simulink model "ramp06"  (Simulink 10.0)
settings: Solver=VariableStepAuto  StartTime=0.0  StopTime=50  FixedStep=1/1000  RelTol=1e-3
model workspace (MAT data in the model file):
  A = [1  -0.0098; 0  1]
  B = [0.001; 0]
  P0 = [1000000  0; 0  1000000]
  P1 = [1000000  0  0  0  0  0  0  0  0  0  0  0  0  0  0  0  0  0  0  0; 0  1000000  0  0  0  0  0  0  0  0  0  0  0  0  0  0  0  0  0  0; 0  0  1000000  0  0  0  0  0  0  0  0  0  0  0  0  0  0  0  0  0; 0  0  0  1000000  0  0  0  0  0  0  0  0  0  0  0  0  0  0  0  0; 0  0  0  0  1000000  0  0  0  0  0  0  0  0  0  0  0  0  0  0  0; 0  0  0  0  0  1000000  0  0  0  0  0  0  0  0  0  0  0  0  0  0; 0  0  0  0  0  0  1000000  0  0  0  0  0  0  0  0  0  0  0  0  0; 0  0  0  0  0  0  0  1000000  0  0  0  0  0  0  0  0  0  0  0  0; 0  0  0  0  0  0  0  0  1000000  0  0  0  0  0  0  0  0  0  0  0; 0  0  0  0  0  0  0  0  0  1000000  0  0  0  0  0  0  0  0  0  0; 0  0  0  0  0  0  0  0  0  0  1000000  0  0  0  0  0  0  0  0  0; 0  0  0  0  0  0  0  0  0  0  0  1000000  0  0  0  0  0  0  0  0; 0  0  0  0  0  0  0  0  0  0  0  0  1000000  0  0  0  0  0  0  0; 0  0  0  0  0  0  0  0  0  0  0  0  0  1000000  0  0  0  0  0  0; 0  0  0  0  0  0  0  0  0  0  0  0  0  0  1000000  0  0  0  0  0; 0  0  0  0  0  0  0  0  0  0  0  0  0  0  0  1000000  0  0  0  0; 0  0  0  0  0  0  0  0  0  0  0  0  0  0  0  0  1000000  0  0  0; 0  0  0  0  0  0  0  0  0  0  0  0  0  0  0  0  0  1000000  0  0; 0  0  0  0  0  0  0  0  0  0  0  0  0  0  0  0  0  0  1000000  0; 0  0  0  0  0  0  0  0  0  0  0  0  0  0  0  0  0  0  0  1000000]
  P2 = 1000000
  X0 = [14; 0]
  dett = 0.001
  f = 0.0038
  g : num (value not decoded)
libraries: simulink x1, Solver_SF x1
settings Model: Creator=JHD  LastModifiedBy=JHD  OrderedModelArguments=off
settings DataIOCC: SaveFormat=Dataset  ReturnWorkspaceOutputs=on
settings OptimizationCC: LifeSpan=auto
settings DebuggingCC: UnderspecifiedInitializationDetection=Simplified  MergeDetectMultiDrivingBlocksExec=error  SFUnexpectedBacktrackingDiag=error  SFNoUnconditionalDefaultTransitionDiag=error  SFExecutionAtInitializationDiag=warning  ArithmeticOperatorsInVariantConditions=error
settings HardwareCC: ProdBitPerPointer=64  ProdBitPerSizeT=64  ProdBitPerPtrDiffT=64  ProdLargestAtomicFloat=Float  ProdIntDivRoundTo=Zero  ProdEndianess=LittleEndian  ProdWordSize=64  ProdHWDeviceType=Intel->x86-64 (Windows64)
settings ModelReferenceCC: PropagateSignalLabelsOutOfModel=on
settings SFSimCC: SimUseLocalCustomCode=on  CustomCodeUndefinedFunction=FilterOut
settings RTWCC: RTWUseLocalCustomCode=on
settings CodeAppCC: StateflowObjectComments=off
settings GRTTargetCC: TargetLangStandard=C99 (ISO)  CombineOutputUpdateFcns=on  GRTInterface=off
settings ConfigComp: CovMetricSettings=dwe  CovHtmlReporting=off  CovSaveCumulativeToWorkspaceVar=off  CovSaveSingleToWorkspaceVar=off

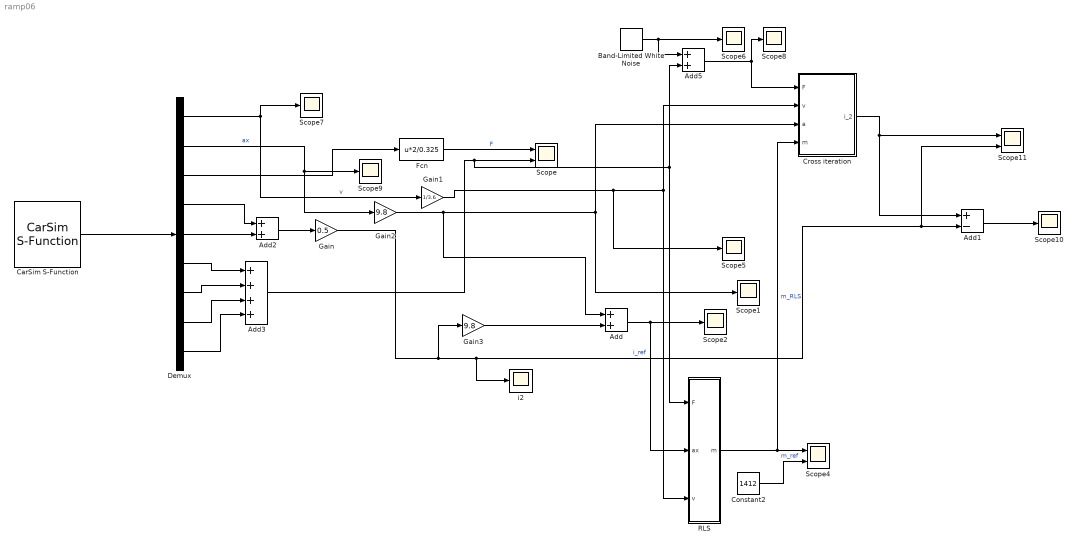
== system ramp06 ==
  Add : Sum
  Add1 : Sum  Inputs=+-
  Add2 : Sum
  Add3 : Sum  Inputs=4
  Add5 : Sum
  Band-Limited White Noise : simulink/Sources/Band-Limited White Noise  Cov=[10]  Ts=0.1  seed=[23341]
  CarSim S-Function : Solver_SF/CarSim S-Function  Priority=1  SIMFILE=simfile.sim
  Constant2 : Constant  Value=1412
  Cross iteration : Subsystem
  Demux : Demux  Outputs=9
  Fcn : Fcn  Expr=u*2/0.325
  Gain : Gain  Gain=0.5
  Gain1 : Gain  Gain=1/3.6
  Gain2 : Gain  Gain=9.8
  Gain3 : Gain  Gain=9.8
  RLS : Subsystem
  Scope : Scope  NumInputPorts=2
  Scope{1..2,5..10} (8 alike) : Scope
  Scope11 : Scope  NumInputPorts=2
  Scope4 : Scope  NumInputPorts=2
  i2 : Scope
  wires:
  CarSim S-Function/1 -> Demux/1
  Demux/2 -> Scope9/1, Gain2/1  "ax"
  Demux/1 -> Scope7/1, Gain1/1  "v"
  Gain/1 -> Gain3/1, i2/1, Scope11/2, Add1/2  "i_ref"
  Demux/4 -> Add2/1
  Demux/5 -> Add2/2
  Add2/1 -> Gain/1
  Constant2/1 -> Scope4/2  "m_ref"
  Demux/3 -> Fcn/1
  Demux/6 -> Add3/1
  Demux/7 -> Add3/2
  Demux/8 -> Add3/3
  Demux/9 -> Add3/4
  Fcn/1 -> Scope/1  "F"
  Cross iteration/1(i_2) -> Scope11/1, Add1/1
  Add3/1 -> Add5/2, RLS/1(F), Scope/2
  Gain3/1 -> Add/2
  Add/1 -> RLS/2(ax), Scope2/1
  RLS/1(m) -> Cross iteration/4(m), Scope4/1  "m_RLS"
  Add1/1 -> Scope10/1
  Gain2/1 -> Cross iteration/3(a), Scope1/1, Add/1
  Gain1/1 -> Scope5/1, RLS/3(v), Cross iteration/2(v)
  Band-Limited White Noise/1 -> Add5/1, Scope6/1
  Add5/1 -> Scope8/1, Cross iteration/1(F)

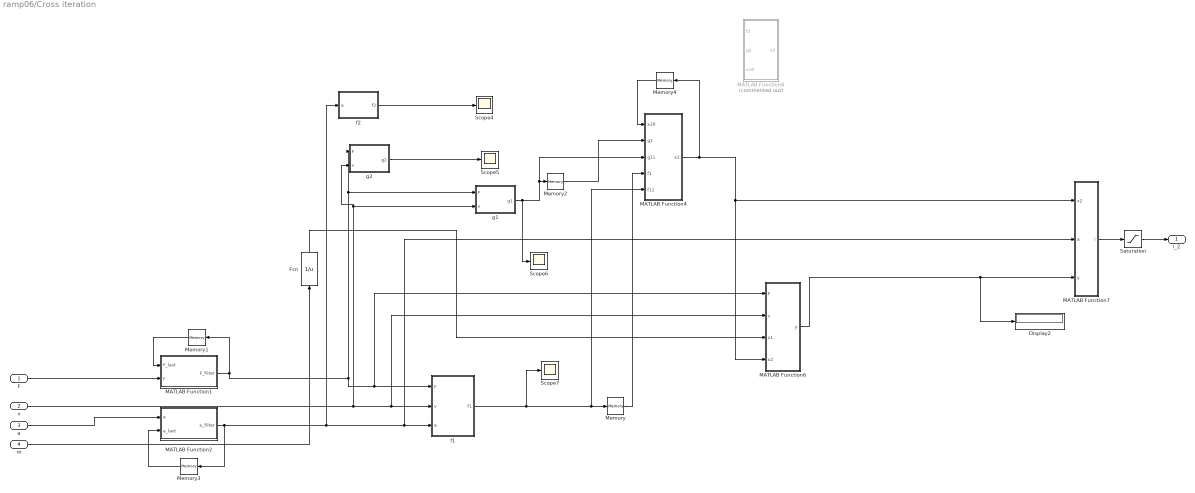
== system ramp06/Cross iteration ==
  F : Inport
  v : Inport  Port=2
  a : Inport  Port=3
  m : Inport  Port=4
  Display2 : Display
  Fcn : Fcn  Expr=1/u
  MATLAB Function1 : MATLAB Function  TreatAsAtomicUnit=on
  MATLAB Function2 : MATLAB Function  TreatAsAtomicUnit=on
  MATLAB Function4 : MATLAB Function  TreatAsAtomicUnit=on
  MATLAB Function6 : MATLAB Function  TreatAsAtomicUnit=on
  MATLAB Function7 : MATLAB Function  TreatAsAtomicUnit=on
  MATLAB Function8 : MATLAB Function  Commented=on  TreatAsAtomicUnit=on
  Memory{,1..3} (4 alike) : Memory
  Memory4 : Memory  InitialCondition=0.1
  Saturation : Saturate
  Scope{4..7} (4 alike) : Scope
  f1 : MATLAB Function  TreatAsAtomicUnit=on
  f2 : MATLAB Function  TreatAsAtomicUnit=on
  g1 : MATLAB Function  TreatAsAtomicUnit=on
  g2 : MATLAB Function  TreatAsAtomicUnit=on
  i_2 : Outport
  wires:
  F/1 -> MATLAB Function1/2(F)
  a/1 -> MATLAB Function2/1(a)
  v/1 -> f1/2(v), MATLAB Function6/2(v), g1/2(v), g2/2(v)
  f1/1(f1) -> Scope7/1, MATLAB Function4/5(f11), Memory/1
  g1/1(g1) -> Scope6/1, MATLAB Function4/3(g11), Memory2/1
  MATLAB Function6/1(y) -> Display2/1, MATLAB Function7/3(y)
  Memory/1 -> MATLAB Function4/4(f1)
  Memory2/1 -> MATLAB Function4/2(g1)
  f2/1(f2) -> Scope4/1
  g2/1(g2) -> Scope5/1
  m/1 -> Fcn/1
  Fcn/1 -> MATLAB Function6/3(x1)
  MATLAB Function4/1(x2) -> MATLAB Function7/1(x2), MATLAB Function6/4(x2), Memory4/1
  MATLAB Function7/1(i) -> Saturation/1
  MATLAB Function1/1(F_filter) -> f1/1(F), MATLAB Function6/1(F), g1/1(F), g2/1(F), Memory1/1
  Memory1/1 -> MATLAB Function1/1(F_last)
  MATLAB Function2/1(a_filter) -> Memory3/1, f1/3(a), MATLAB Function7/2(a), f2/1(a)
  Memory3/1 -> MATLAB Function2/2(a_last)
  Saturation/1 -> i_2/1
  Memory4/1 -> MATLAB Function4/1(x20)

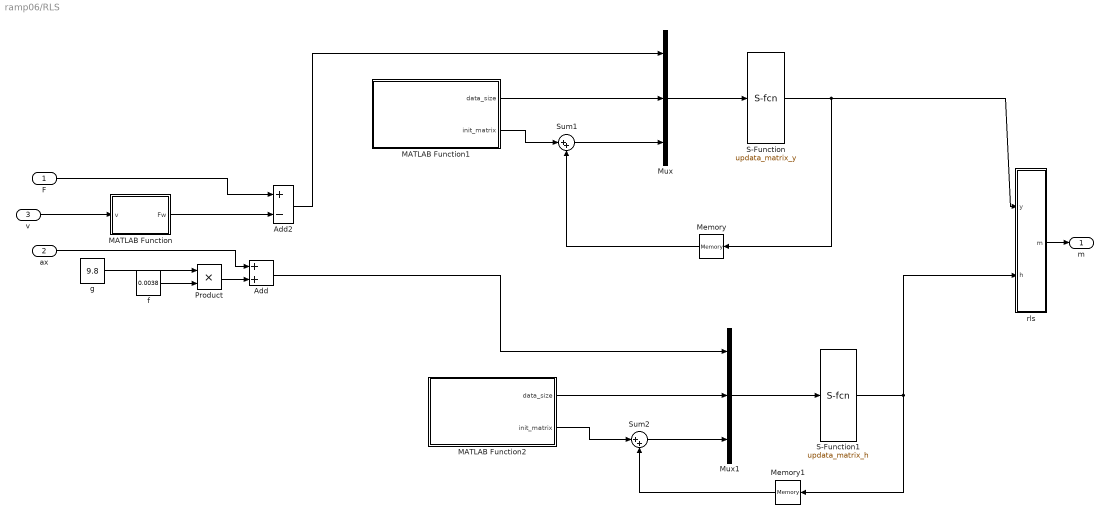
== system ramp06/RLS ==
  F : Inport
  ax : Inport  Port=2
  v : Inport  Port=3
  Add : Sum
  Add2 : Sum  Inputs=+-
  MATLAB Function : MATLAB Function  TreatAsAtomicUnit=on
  MATLAB Function1 : MATLAB Function  TreatAsAtomicUnit=on
  MATLAB Function2 : MATLAB Function  TreatAsAtomicUnit=on
  Memory : Memory
  Memory1 : Memory
  Mux : Mux  Inputs=3
  Mux1 : Mux  Inputs=3
  Product : Product
  S-Function : S-Function  FunctionName=updata_matrix_y  SFunctionDeploymentMode=off  EnableBusSupport=off
  S-Function1 : S-Function  FunctionName=updata_matrix_h  SFunctionDeploymentMode=off  EnableBusSupport=off
  Sum1 : Sum  Inputs=|++
  Sum2 : Sum  Inputs=|++
  f : Constant  Value=0.0038
  g : Constant  Value=9.8
  rls : Subsystem
  m : Outport
  wires:
  F/1 -> Add2/1
  g/1 -> Product/1
  Product/1 -> Add/2
  f/1 -> Product/2
  MATLAB Function/1(Fw) -> Add2/2
  ax/1 -> Add/1
  rls/1(m) -> m/1
  v/1 -> MATLAB Function/1(v)
  MATLAB Function1/1(data_size) -> Mux/2
  Memory/1 -> Sum1/2
  Mux1/1 -> S-Function1/1
  Mux/1 -> S-Function/1
  MATLAB Function2/1(data_size) -> Mux1/2
  Sum1/1 -> Mux/3
  S-Function/1 -> Memory/1, rls/1(y)
  S-Function1/1 -> rls/2(h), Memory1/1
  Sum2/1 -> Mux1/3
  Memory1/1 -> Sum2/2
  Add2/1 -> Mux/1
  Add/1 -> Mux1/1
  MATLAB Function2/2(init_matrix) -> Sum2/1
  MATLAB Function1/2(init_matrix) -> Sum1/1

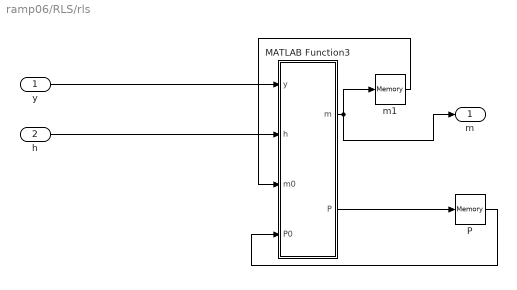
== system ramp06/RLS/rls ==
  y : Inport
  h : Inport  Port=2
  MATLAB Function3 : MATLAB Function  TreatAsAtomicUnit=on
  P : Memory  InitialCondition=P1
  m1 : Memory  InitialCondition=1000  InheritSampleTime=on  LinearizeAsDelay=on
  m : Outport
  wires:
  MATLAB Function3/2(P) -> P/1
  MATLAB Function3/1(m) -> m/1, m1/1
  m1/1 -> MATLAB Function3/3(m0)
  P/1 -> MATLAB Function3/4(P0)
  y/1 -> MATLAB Function3/1(y)
  h/1 -> MATLAB Function3/2(h)

== matlab function Cross iteration/MATLAB Function1 ==
  data: F_last input double; F_filter output double; F input double
function F_filter = fcn(F_last,F)

k=0.1;
F_filter = F*k+F_last*(1-k);

== matlab function Cross iteration/MATLAB Function2 ==
  data: a input double; a_last input double; a_filter output double
function a_filter = fcn(a,a_last)

k=0.1;
a_filter = a*k+a_last*(1-k);

== matlab function RLS/MATLAB Function2 ==
  data: data_size output double; init_matrix output double
function [data_size,init_matrix]= prediction_size( )

init_matrix=zeros(20,1);%x.y，phai,vl,vr初始,,,,修改历史数据集大小还需要修改sfunction输出个数
data_size=20;

== matlab function RLS/rls/MATLAB Function3 ==
  data: y input double; m output double; h input double; m0 input double; P0 input double; P output double
function [m,P] = fcn(y,h,m0,P0)

na=1.005;

K = P0*h/(na+h'*P0*h);
I=eye(20);
P = 1/na*(I-K*h')*P0;
m = m0+K'*(y-m0*h);

== matlab function RLS/MATLAB Function ==
  data: v input double; Fw output double
function Fw = fcn(v)

Cd=0.3;
rou=1.206;
A=2.2;
Fw = Cd*rou*A/2*v*v;

== matlab function Cross iteration/f1 ==
  data: F input double; f1 output double; v input double; a input double
function f1 = fcn(F,v,a)

Cd=0.3;
rou=1.206;
A=2.2;
Fw = Cd*rou*A/2*v*v;
f1 = a/(F-Fw);

== matlab function Cross iteration/f2 ==
  data: a input double; f2 output double
function f2 = fcn(a)

g=9.8;
f=0.0038;

f2 = a/g/sqrt(1+f*f);

== matlab function Cross iteration/g1 ==
  data: F input double; g1 output double; v input double
function g1 = fcn(F,v)

g=9.8;
f=0.0038;
Cd=0.3;
rou=1.206;
A=2.2;
Fw = Cd*rou*A/2*v*v;


g1 = g*sqrt(1+f*f)/(F-Fw);

== matlab function Cross iteration/g2 ==
  data: F input double; g2 output double; v input double
function g2  = fcn(F,v)

g=9.8;
f=0.0038;
Cd=0.3;
rou=1.206;
A=2.2;
Fw = Cd*rou*A/2*v*v;

g2 = (F-Fw)/g/sqrt(1+f*f);

== matlab function Cross iteration/MATLAB Function4 ==
  data: x20 input double; x2 output double; g1 input double; g11 input double; f1 input double; f11 input double
function x2 = fcn(x20,g1,g11,f1,f11)

x2 = g1*x20/g11-(f1-f11)/g11;

== matlab function Cross iteration/MATLAB Function6 ==
  data: F input double; y output double; v input double; x1 input double; x2 input double
function y = fcn(F,v,x1,x2)

g=9.8;
f=0.0038;
Cd=0.3;
rou=1.206;
A=2.2;
Fw = Cd*rou*A/2*v*v;

fai1=F-Fw;
fai2=-g*sqrt(1+f*f);

y = fai1*x1+fai2*x2;

== matlab function Cross iteration/MATLAB Function7 ==
  data: x2 input double; a input double; y input double; i output double
function i  = fcn(x2,a,y)

g=9.8;
f=0.0038;
fai2=-g*sqrt(1+f*f);
x22=x2+1/fai2*(a-y);
i=tan(x22-atan(f));

== matlab function Cross iteration/MATLAB Function8 ==
  data: f2 input double; x2 output double; g2 input double; x10 input double
function x2 = fcn(f2,g2,x10)

x2 = g2*x10-f2;

== matlab function RLS/MATLAB Function1 ==
  data: data_size output double; init_matrix output double
function [data_size,init_matrix]= prediction_size( )

init_matrix=zeros(20,1);%x.y，phai,vl,vr初始,,,,修改历史数据集大小还需要修改sfunction输出个数
data_size=20;
